simulink model "Cycle_model"  (R2024b)
settings: Solver=FixedStepAuto  StartTime=0.0  StopTime=300  FixedStep=0.01  RelTol=1e-3
InitFcn:
  | load matlab.mat
StopFcn:
  | startLoc = get_param(bdroot, 'ModelWorkspace').getVariable('startLoc');
  | assignin('base', 'startLoc', startLoc);
  | 
  | goalLoc = get_param(bdroot, 'ModelWorkspace').getVariable('goalLoc');
  | assignin('base', 'goalLoc', goalLoc);
  | 
  | InitState = get_param(bdroot, 'ModelWorkspace').getVariable('InitState');
  | assignin('base', 'InitState', InitState);
  | 
  | visualizador_datos_sim
model workspace (MAT data in the model file):
  InitState = [5 5 3.14159265359]
  Ts = 0.01
  goalLoc = [13 7]
  speed_range = [-8 8]
  startLoc = [5 5]
values from neighbouring files (symbols this model uses):
  simpleMap = [1 1 1 1 1 1 1 1 1 1 1 1 ... (702 elements, 26x27)]    [matlab.mat]
undefined symbols (not defined in the file or in its folder): dspblkCoreblockFVToolHelper, gcbh
libraries: simulink x5, slpidlib x2, robotmobilelib x1, robotalgslib x1
settings Model: Creator=Andres  LastModifiedBy=Andres
settings OptimizationCC: DefaultParameterBehavior=Inlined  GainParamInheritBuiltInType=on  UseFloatMulNetSlope=on  OptimizeBlockIOStorage=off
settings RTWCC: BuildConfiguration=Debug
settings CodeAppCC: ForceParamTrailComments=on  MATLABSourceComments=on

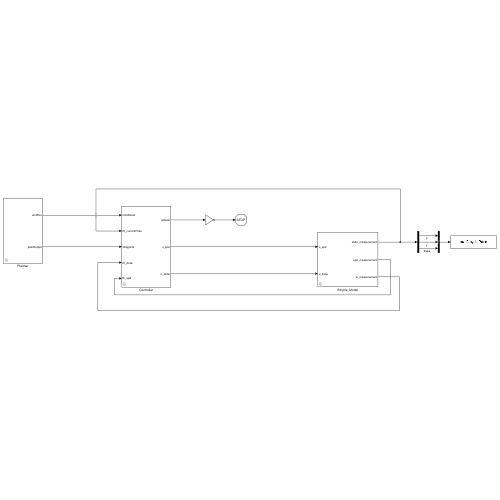
[thumbnail: Simulink's stored preview of the top-level diagram]
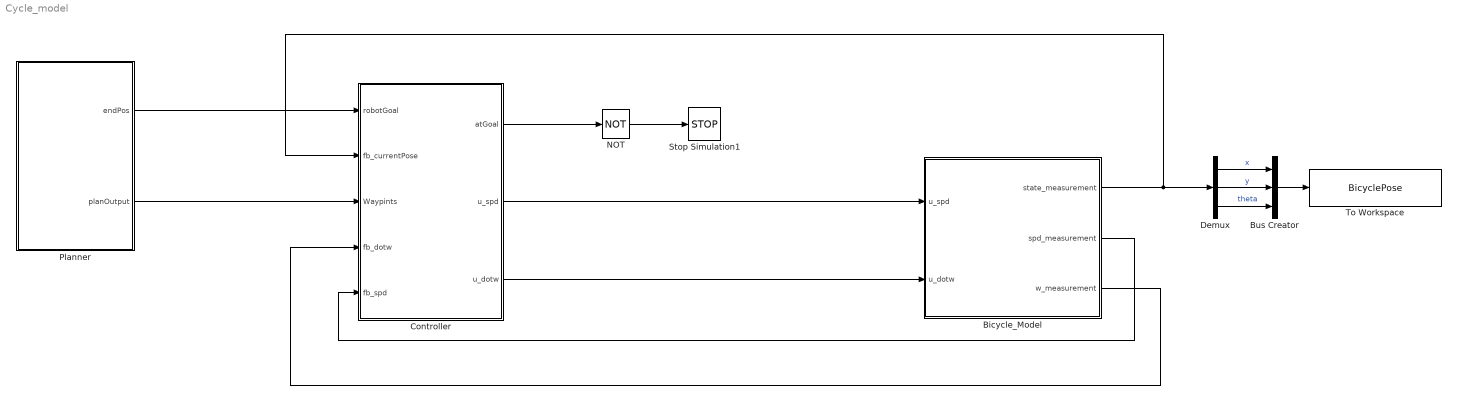
== system Cycle_model ==
  Bicycle_Model : Subsystem  mask{WheelBase=1, InitialState=InitState, MaxSteeringAngle=pi/4, VehicleSpeedRange=speed_range, tau_rad=0.2, tau_spd=3}
      mask prompts: WheelBase "robotics:robotslmobile:sharedblockmask:WheelBasePrompt"; InitialState "robotics:robotslmobile:sharedblockmask:InitialStatePrompt"; MaxSteeringAngle "robotics:robotslmobile:sharedblockmask:MaxSteeringAnglePrompt"; VehicleSpeedRange "robotics:robotslmobile:sharedblockmask:VehicleSpeedRangePrompt"; tau_rad "Time from 0 rad to max steering angle (s)"; tau_spd "Time form 0 m/s to max speed (s)"
      mask TypeOptions WheelBase: Model/WheelBase
      mask TypeOptions InitialState: Model/InitialState
      mask TypeOptions MaxSteeringAngle: Model/MaxSteeringAngle
      mask TypeOptions VehicleSpeedRange: Model/VehicleSpeedRange
      mask TypeOptions tau_rad: Model/tau_rad
      mask TypeOptions tau_spd: Model/tau_spd
      mask DialogControl DescGroupVar Prompt: Bicycle Model (mask)
      mask DialogControl WheelBase Prompt: Wheel base (m):
      mask DialogControl InitialState Prompt: Initial state:
      mask DialogControl MaxSteeringAngle Prompt: Maximum steering angle (rad):
      mask DialogControl VehicleSpeedRange Prompt: Vehicle speed range (m/s):
  Bus Creator : BusCreator  Inputs=3
  Controller : Subsystem  mask{Kp_dotw=1, Ki_dotw=0.01, Kp_lin=0.1, Ki_lin=0.1, DesiredLinearVelocity=2, LookaheadDistance=0.5, MaxAngularVelocity=7}
      mask prompts: Kp_dotw "Kp"; Ki_dotw "Ki"; Kp_lin "Kp"; Ki_lin "Ki"; DesiredLinearVelocity "Desired linear velocity (m/s):"; LookaheadDistance "Lookahead distance (m):"; MaxAngularVelocity "Maximum angular velocity (rad/s):"
      mask TypeOptions DesiredLinearVelocity: Pure Pursuit/DesiredLinearVelocity
      mask TypeOptions LookaheadDistance: Pure Pursuit/LookaheadDistance
      mask TypeOptions MaxAngularVelocity: Pure Pursuit/MaxAngularVelocity
      mask DialogControl DescGroupVar Prompt: Controller (mask)
      mask DialogControl ParameterGroupVar Prompt: PI angular velocity
      mask DialogControl ParameterGroupVar_copy Prompt: PI linear velocity
  Demux : Demux  Outputs=3
  NOT : Logic  Operator=NOT  IconShape=distinctive  AllPortsSameDT=off  OutDataTypeStr=boolean
  Planner : Subsystem  mask{startLoc=startLoc, goalLoc=goalLoc, simpleMap=simpleMap}
      mask prompts: startLoc "Start Location [x y]"; goalLoc "Goal Location"; simpleMap "Map"
      mask DialogControl DescGroupVar Prompt: Planner (mask)
  Stop Simulation1 : Stop
  To Workspace : ToWorkspace  VariableName=BicyclePose  SaveFormat=Timeseries  SampleTime=-1
  wires:
  NOT/1 -> Stop Simulation1/1
  Demux/1 -> Bus Creator/1  "x"
  Demux/2 -> Bus Creator/2  "y"
  Demux/3 -> Bus Creator/3  "theta"
  Bus Creator/1 -> To Workspace/1
  Bicycle_Model/1(state_measurement) -> Demux/1, Controller/2(fb_currentPose)
  Bicycle_Model/2(spd_measurement) -> Controller/5(fb_spd)
  Planner/1(endPos) -> Controller/1(robotGoal)
  Planner/2(planOutput) -> Controller/3(Waypints)
  Bicycle_Model/3(w_measurement) -> Controller/4(fb_dotw)
  Controller/1(atGoal) -> NOT/1
  Controller/2(u_spd) -> Bicycle_Model/1(u_spd)
  Controller/3(u_dotw) -> Bicycle_Model/2(u_dotw)

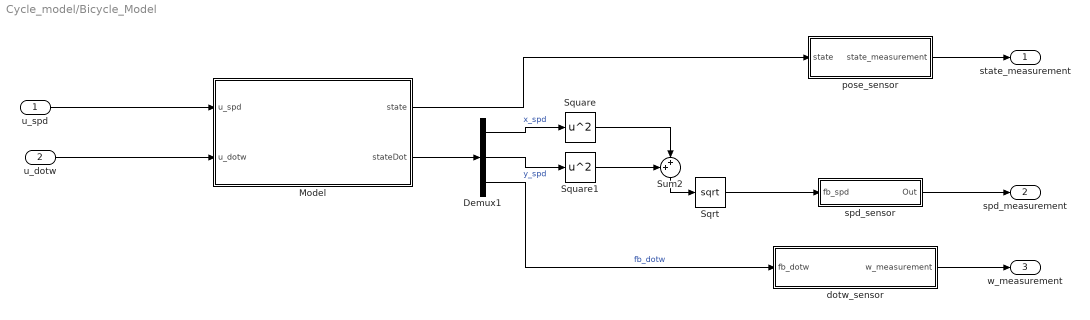
== system Cycle_model/Bicycle_Model ==
  u_spd : Inport
  u_dotw : Inport  Port=2
  Demux1 : Demux  Outputs=3
  Model : Subsystem  mask{InitialState=InitialState, WheelBase=WheelBase, VehicleSpeedRange=VehicleSpeedRange, MaxSteeringAngle=MaxSteeringAngle, tau_spd=tau_spd, tau_rad=tau_rad}
      mask prompts: InitialState "robotics:robotslmobile:sharedblockmask:InitialStatePrompt"; WheelBase "robotics:robotslmobile:sharedblockmask:WheelBasePrompt"; VehicleSpeedRange "robotics:robotslmobile:sharedblockmask:VehicleSpeedRangePrompt"; MaxSteeringAngle "robotics:robotslmobile:sharedblockmask:MaxSteeringAnglePrompt"; tau_spd "Time form 0 m/s to max speed (s)"; tau_rad "Time from 0 rad to max steering angle (s)"
      mask TypeOptions InitialState: Bicycle Kinematic Model/InitialState
      mask TypeOptions WheelBase: Bicycle Kinematic Model/WheelBase
      mask TypeOptions VehicleSpeedRange: Bicycle Kinematic Model/VehicleSpeedRange
      mask TypeOptions MaxSteeringAngle: Bicycle Kinematic Model/MaxSteeringAngle
      mask DialogControl ParameterGroupVar Prompt: Bicycle Parameters
      mask DialogControl InitialState Prompt: Initial state:
      mask DialogControl WheelBase Prompt: Wheel base (m):
      mask DialogControl VehicleSpeedRange Prompt: Vehicle speed range (m/s):
      mask DialogControl MaxSteeringAngle Prompt: Maximum steering angle (rad):
  Sqrt : Sqrt
  Square : Math  Operator=square
  Square1 : Math  Operator=square
  Sum2 : Sum  Inputs=++|
  dotw_sensor : Subsystem
  pose_sensor : Subsystem
  spd_sensor : Subsystem  mask{NsPw=0.0000004, Nhz=1000}
      mask prompts: NsPw "Noise Power"; Nhz "Noise Hz"
  state_measurement : Outport
  spd_measurement : Outport  Port=2
  w_measurement : Outport  Port=3
  wires:
  Square1/1 -> Sum2/1
  Demux1/1 -> Square/1  "x_spd"
  Sqrt/1 -> spd_sensor/1(fb_spd)
  Demux1/2 -> Square1/1  "y_spd"
  Model/2(stateDot) -> Demux1/1
  Square/1 -> Sum2/2
  Sum2/1 -> Sqrt/1
  u_dotw/1 -> Model/2(u_dotw)
  u_spd/1 -> Model/1(u_spd)
  Demux1/3 -> dotw_sensor/1(fb_dotw)  "fb_dotw"
  Model/1(state) -> pose_sensor/1(state)
  pose_sensor/1(state_measurement) -> state_measurement/1
  spd_sensor/1(Out) -> spd_measurement/1
  dotw_sensor/1(w_measurement) -> w_measurement/1

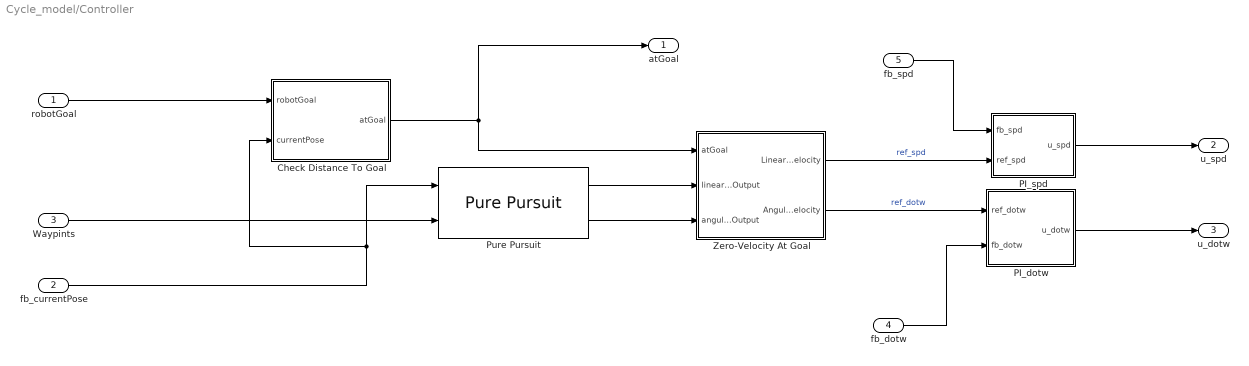
== system Cycle_model/Controller ==
  robotGoal : Inport
  fb_currentPose : Inport  Port=2
  Waypints : Inport  Port=3
  fb_dotw : Inport  Port=4
  fb_spd : Inport  Port=5
  Check Distance To Goal : Subsystem
  PI_dotw : Subsystem
  PI_spd : Subsystem
  Pure Pursuit : robotalgslib/Pure Pursuit  DesiredLinearVelocityPort=off  DesiredLinearVelocity=DesiredLinearVelocity  MaxAngularVelocity=MaxAngularVelocity  LookaheadDistancePort=off  LookaheadDistance=LookaheadDistance  TargetDirPort=off  SimulateUsing=Code generation
      settings: LibrarySourceBlock=robotmobilelib/Pure Pursuit
  Zero-Velocity At Goal : Subsystem
  atGoal : Outport
  u_spd : Outport  Port=2
  u_dotw : Outport  Port=3
  wires:
  Pure Pursuit/2 -> Zero-Velocity At Goal/3(angularVelocityOutput)
  Pure Pursuit/1 -> Zero-Velocity At Goal/2(linearVelocityOutput)
  fb_currentPose/1 -> Pure Pursuit/1, Check Distance To Goal/2(currentPose)
  Check Distance To Goal/1(atGoal) -> atGoal/1, Zero-Velocity At Goal/1(atGoal)
  fb_spd/1 -> PI_spd/1(fb_spd)
  fb_dotw/1 -> PI_dotw/2(fb_dotw)
  robotGoal/1 -> Check Distance To Goal/1(robotGoal)
  Waypints/1 -> Pure Pursuit/2
  Zero-Velocity At Goal/2(Angular Velocity) -> PI_dotw/1(ref_dotw)  "ref_dotw"
  PI_dotw/1(u_dotw) -> u_dotw/1
  PI_spd/1(u_spd) -> u_spd/1
  Zero-Velocity At Goal/1(Linear Velocity) -> PI_spd/2(ref_spd)  "ref_spd"

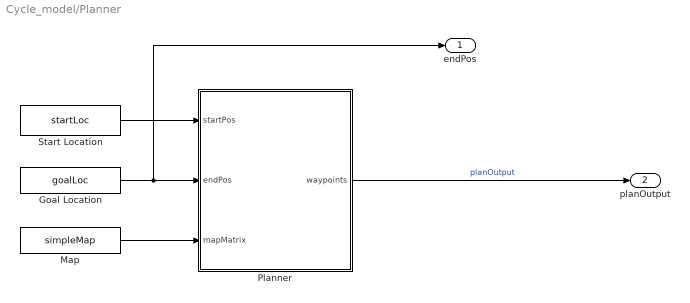
== system Cycle_model/Planner ==
  Goal Location : Constant  Value=goalLoc
  Map : Constant  Value=simpleMap
  Planner : MATLAB Function  TreatAsAtomicUnit=on
  Start Location : Constant  Value=startLoc
  endPos : Outport
  planOutput : Outport  Port=2
  wires:
  Goal Location/1 -> endPos/1, Planner/2(endPos)
  Start Location/1 -> Planner/1(startPos)
  Map/1 -> Planner/3(mapMatrix)
  Planner/1(waypoints) -> planOutput/1  "planOutput"

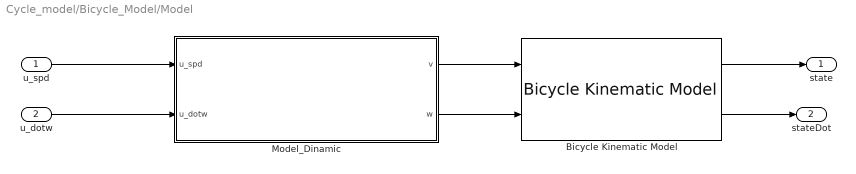
== system Cycle_model/Bicycle_Model/Model ==
  u_spd : Inport
  u_dotw : Inport  Port=2
  Bicycle Kinematic Model : robotmobilelib/Bicycle Kinematic Model  VehicleInputs=Vehicle Speed & Heading Angular Velocity  WheelBase=WheelBase  VehicleSpeedRange=VehicleSpeedRange  MaxSteeringAngle=MaxSteeringAngle  InitialState=InitialState  SimulateUsing=Interpreted execution
  Model_Dinamic : Subsystem
  state : Outport
  stateDot : Outport  Port=2
  wires:
  Bicycle Kinematic Model/1 -> state/1
  Bicycle Kinematic Model/2 -> stateDot/1
  u_spd/1 -> Model_Dinamic/1(u_spd)
  Model_Dinamic/1(v) -> Bicycle Kinematic Model/1
  Model_Dinamic/2(w) -> Bicycle Kinematic Model/2
  u_dotw/1 -> Model_Dinamic/2(u_dotw)

== system Cycle_model/Bicycle_Model/dotw_sensor ==
  fb_dotw : Inport
  Low-Pass Filter1 : TransferFcn  Denominator=[0.05 1]
  Zero-Order Hold3 : ZeroOrderHold  SampleTime=Ts
  w_measurement : Outport
  wires:
  Low-Pass Filter1/1 -> Zero-Order Hold3/1
  Zero-Order Hold3/1 -> w_measurement/1
  fb_dotw/1 -> Low-Pass Filter1/1

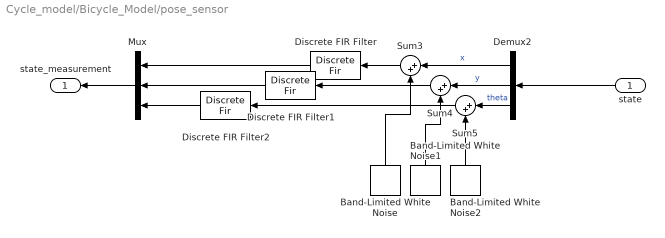
== system Cycle_model/Bicycle_Model/pose_sensor ==
  state : Inport
  Band-Limited White Noise : simulink/Sources/Band-Limited White Noise  Cov=[0.0004]  Ts=0.1  seed=123
  Band-Limited White Noise1 : simulink/Sources/Band-Limited White Noise  Cov=[0.0004]  Ts=0.1  seed=456
  Band-Limited White Noise2 : simulink/Sources/Band-Limited White Noise  Cov=0.000025  Ts=0.1  seed=789
  Demux2 : Demux  Outputs=3
  Discrete FIR Filter : DiscreteFir  LoadFcn=dspblkCoreblockFVToolHelper(gcbh,'load');  Coefficients="[0.0625,  0.2500,  0.3750,  0.2500,  0.0625]"  InitialStates=5
      settings: CopyFcn=dspblkCoreblockFVToolHelper(gcbh,'copy');  DeleteFcn=dspblkCoreblockFVToolHelper(gcbh,'close');  ModelCloseFcn=dspblkCoreblockFVToolHelper(gcbh,'close');  PreSaveFcn=dspblkCoreblockFVToolHelper(gcbh,'presave');  PostSaveFcn=dspblkCoreblockFVToolHelper(gcbh,'postsave');  CloseFcn=dspblkCoreblockFVToolHelper(gcbh,'close');
  Discrete FIR Filter1 : DiscreteFir  LoadFcn=dspblkCoreblockFVToolHelper(gcbh,'load');  Coefficients="[0.0625,  0.2500,  0.3750,  0.2500,  0.0625]"  InitialStates=5
      settings: CopyFcn=dspblkCoreblockFVToolHelper(gcbh,'copy');  DeleteFcn=dspblkCoreblockFVToolHelper(gcbh,'close');  ModelCloseFcn=dspblkCoreblockFVToolHelper(gcbh,'close');  PreSaveFcn=dspblkCoreblockFVToolHelper(gcbh,'presave');  PostSaveFcn=dspblkCoreblockFVToolHelper(gcbh,'postsave');  CloseFcn=dspblkCoreblockFVToolHelper(gcbh,'close');
  Discrete FIR Filter2 : DiscreteFir  LoadFcn=dspblkCoreblockFVToolHelper(gcbh,'load');  Coefficients="[0.0625,  0.2500,  0.3750,  0.2500,  0.0625]"  InitialStates=pi
      settings: CopyFcn=dspblkCoreblockFVToolHelper(gcbh,'copy');  DeleteFcn=dspblkCoreblockFVToolHelper(gcbh,'close');  ModelCloseFcn=dspblkCoreblockFVToolHelper(gcbh,'close');  PreSaveFcn=dspblkCoreblockFVToolHelper(gcbh,'presave');  PostSaveFcn=dspblkCoreblockFVToolHelper(gcbh,'postsave');  CloseFcn=dspblkCoreblockFVToolHelper(gcbh,'close');
  Mux : Mux  Inputs=3
  Sum3 : Sum  Inputs=|++
  Sum4 : Sum  Inputs=|++
  Sum5 : Sum  Inputs=|++
  state_measurement : Outport
  wires:
  Sum4/1 -> Discrete FIR Filter1/1
  Band-Limited White Noise/1 -> Sum3/2
  Sum5/1 -> Discrete FIR Filter2/1
  Discrete FIR Filter/1 -> Mux/1
  Demux2/2 -> Sum4/1  "y"
  Band-Limited White Noise1/1 -> Sum4/2
  Discrete FIR Filter1/1 -> Mux/2
  Band-Limited White Noise2/1 -> Sum5/2
  Discrete FIR Filter2/1 -> Mux/3
  Demux2/3 -> Sum5/1  "theta"
  Sum3/1 -> Discrete FIR Filter/1
  Demux2/1 -> Sum3/1  "x"
  Mux/1 -> state_measurement/1
  state/1 -> Demux2/1

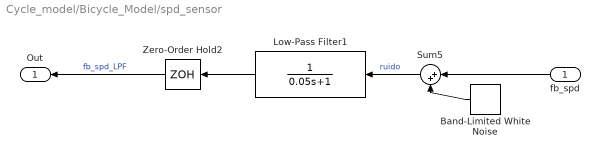
== system Cycle_model/Bicycle_Model/spd_sensor ==
  fb_spd : Inport
  Band-Limited White Noise : simulink/Sources/Band-Limited White Noise  Cov=[NsPw]  Ts=Ts  seed=[23341]
  Low-Pass Filter1 : TransferFcn  Denominator=[0.05 1]
  Sum5 : Sum  Inputs=|++
  Zero-Order Hold2 : ZeroOrderHold  SampleTime=Ts
  Out : Outport
  wires:
  Low-Pass Filter1/1 -> Zero-Order Hold2/1
  Sum5/1 -> Low-Pass Filter1/1  "ruido"
  Band-Limited White Noise/1 -> Sum5/2
  fb_spd/1 -> Sum5/1
  Zero-Order Hold2/1 -> Out/1  "fb_spd_LPF"

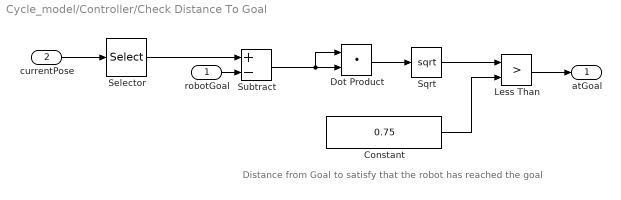
== system Cycle_model/Controller/Check Distance To Goal ==
  note: Distance from Goal to satisfy that the robot has reached the goal
  robotGoal : Inport
  currentPose : Inport  Port=2
  Constant : Constant  Value=0.75
  Dot Product : DotProduct  OutDataTypeStr=Inherit: Inherit via internal rule
  Less Than : RelationalOperator  Operator=>  OutDataTypeStr=boolean  RndMeth=Simplest  InputSameDT=off
  Selector : Selector  InputPortWidth=3  IndexOptions=Index vector (dialog)  Indices=[1 2]  OutputSizes=1
  Sqrt : Sqrt
  Subtract : Sum  Inputs=+-
  atGoal : Outport
  wires:
  robotGoal/1 -> Subtract/2
  Dot Product/1 -> Sqrt/1
  Constant/1 -> Less Than/2
  currentPose/1 -> Selector/1
  Less Than/1 -> atGoal/1
  Sqrt/1 -> Less Than/1
  Subtract/1 -> Dot Product/1, Dot Product/2
  Selector/1 -> Subtract/1

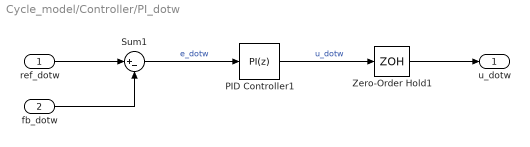
== system Cycle_model/Controller/PI_dotw ==
  ref_dotw : Inport
  fb_dotw : Inport  Port=2
  PID Controller1 : slpidlib/PID Controller  Controller=PI  Form=Parallel  TimeDomain=Discrete-time  UseExternalTs=off  SampleTime=Ts  IntegratorMethod=Forward Euler  FilterMethod=Forward Euler  ControllerParametersSource=internal  P=Kp_dotw  I=Ki_dotw  UseKiTs=off  D=0  UseExternalDerivativeSource=off  N=100  UseFilter=on  TunerSelectOption=Transfer Function Based (PID Tuner App)  InitialConditionSource=internal  InitialConditionForIntegrator=0  InitialConditionForFilter=0  DifferentiatorICPrevScaledInput=0  ExternalReset=none  TrackingMode=off  Kt=1  LimitOutput=on  SatLimitsSource=internal  UpperSaturationLimit=1  LowerSaturationLimit=-1  LinearizeAsGain=off  AntiWindupMode=clamping  Kb=0.01  LimitIntegrator=off  UpperIntegratorSaturationLimit=inf  LowerIntegratorSaturationLimit=-inf  POutMin=[]  POutMax=[]  IOutMin=[]  IOutMax=[]  DOutMin=[]  DOutMax=[]  NOutMin=[]  NOutMax=[]  SumOutMin=[]  SumOutMax=[]  SaturationOutMin=[]  SaturationOutMax=[]  PParamMin=[]  PParamMax=[]  IParamMin=[]  IParamMax=[]  DParamMin=[]  DParamMax=[]  NParamMin=[]  NParamMax=[]  KbParamMin=[]  KbParamMax=[]  KtParamMin=[]  KtParamMax=[]  KbOutMin=[]  KbOutMax=[]  KtOutMin=[]  KtOutMax=[]  IntegratorOutMin=[]  IntegratorOutMax=[]  FilterOutMin=[]  FilterOutMax=[]  SumI1OutMin=[]  SumI1OutMax=[]  SumI2OutMin=[]  SumI2OutMax=[]  SumI3OutMin=[]  SumI3OutMax=[]  SumI4OutMin=[]  SumI4OutMax=[]  SumDOutMin=[]  SumDOutMax=[]  DifferentiatorOutMin=[]  DifferentiatorOutMax=[]  FilterDiffOutCoefMin=[]  FilterDiffOutCoefMax=[]  ReciprocalOutMin=[]  ReciprocalOutMax=[]  SumDenOutMin=[]  SumDenOutMax=[]  SumNumOutMin=[]  SumNumOutMax=[]  DivideOutMin=[]  DivideOutMax=[]  UdiffTsProdOutMin=[]  UdiffTsProdOutMax=[]  NTsProdOutMin=[]  NTsProdOutMax=[]  UintegralTsProdOutMin=[]  UintegralTsProdOutMax=[]  UngainTsProdOutMin=[]  UngainTsProdOutMax=[]  ClampingZeroOutDataTypeStr=Inherit: Inherit via back propagation  ClampingZeroOutMin=[]  ClampingZeroOutMax=[]  FilterDenConstantOutDataTypeStr=Inherit: Inherit via back propagation  FilterDenConstantOutMin=[]  FilterDenConstantOutMax=[]  PCopyOutDataTypeStr=Inherit: Inherit via back propagation  PCopyOutMin=[]  PCopyOutMax=[]  NCopyOutDataTypeStr=Inherit: Inherit via back propagation  NCopyOutMin=[]  NCopyOutMax=[]  IntegratorContinuousStateAttributes=''  IntegratorStateMustResolveToSignalObject=off  IntegratorRTWStateStorageClass=Auto  FilterContinuousStateAttributes=''  FilterStateMustResolveToSignalObject=off  FilterRTWStateStorageClass=Auto  ParallelPVariant=InternalParameters  IdealPVariant=Disabled  IVariant=InternalParameters  DVariant=Disabled  IntegratorVariant=Discrete  SatVariant=Enabled  AWVariant=DiscClampingParallel  PCopyVariant=Disabled  TRVariant=Disabled  FdbkBlocksVariant=Forward  IdealPFdbkVariant=Disabled  SatFdbkVariant=Disabled  DerivativeFilterVariant=Disabled  NVariant=Disabled  NCopyVariant=Disabled_SignalSpec  FilterICVariant=Disabled  IntegratorICVariant=InternalICs  ExternalResetVariant=Disabled  TRSumVariant=Passthrough  SumFdbkVariant=Disabled  SumVariant=Sum_PI  TsampFilterVariant=InternalTs  TsampNgainVariant=Passthrough  TsampIntegralVariant=Disabled_SignalSpec  ExternalSaturationOutDataTypeStr=Inherit: Same as second input  DerivativeSourceVariant=Disabled  PreIntVariant=InternalPreInt
  Sum1 : Sum  Inputs=|+-
  Zero-Order Hold1 : ZeroOrderHold  SampleTime=Ts
  u_dotw : Outport
  wires:
  Sum1/1 -> PID Controller1/1  "e_dotw"
  PID Controller1/1 -> Zero-Order Hold1/1  "u_dotw"
  Zero-Order Hold1/1 -> u_dotw/1
  ref_dotw/1 -> Sum1/1
  fb_dotw/1 -> Sum1/2

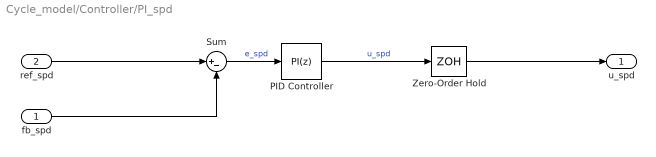
== system Cycle_model/Controller/PI_spd ==
  fb_spd : Inport
  ref_spd : Inport  Port=2
  PID Controller : slpidlib/PID Controller  Controller=PI  Form=Parallel  TimeDomain=Discrete-time  UseExternalTs=off  SampleTime=Ts  IntegratorMethod=Forward Euler  FilterMethod=Forward Euler  ControllerParametersSource=internal  P=Kp_lin  I=Ki_lin  UseKiTs=off  D=0  UseExternalDerivativeSource=off  N=100  UseFilter=on  TunerSelectOption=Transfer Function Based (PID Tuner App)  InitialConditionSource=internal  InitialConditionForIntegrator=0  InitialConditionForFilter=0  DifferentiatorICPrevScaledInput=0  ExternalReset=none  TrackingMode=off  Kt=1  LimitOutput=on  SatLimitsSource=internal  UpperSaturationLimit=1  LowerSaturationLimit=-1  LinearizeAsGain=on  AntiWindupMode=clamping  Kb=0.01  LimitIntegrator=off  UpperIntegratorSaturationLimit=inf  LowerIntegratorSaturationLimit=-inf  POutMin=[]  POutMax=[]  IOutMin=[]  IOutMax=[]  DOutMin=[]  DOutMax=[]  NOutMin=[]  NOutMax=[]  SumOutMin=[]  SumOutMax=[]  SaturationOutMin=[]  SaturationOutMax=[]  PParamMin=[]  PParamMax=[]  IParamMin=[]  IParamMax=[]  DParamMin=[]  DParamMax=[]  NParamMin=[]  NParamMax=[]  KbParamMin=[]  KbParamMax=[]  KtParamMin=[]  KtParamMax=[]  KbOutMin=[]  KbOutMax=[]  KtOutMin=[]  KtOutMax=[]  IntegratorOutMin=[]  IntegratorOutMax=[]  FilterOutMin=[]  FilterOutMax=[]  SumI1OutMin=[]  SumI1OutMax=[]  SumI2OutMin=[]  SumI2OutMax=[]  SumI3OutMin=[]  SumI3OutMax=[]  SumI4OutMin=[]  SumI4OutMax=[]  SumDOutMin=[]  SumDOutMax=[]  DifferentiatorOutMin=[]  DifferentiatorOutMax=[]  FilterDiffOutCoefMin=[]  FilterDiffOutCoefMax=[]  ReciprocalOutMin=[]  ReciprocalOutMax=[]  SumDenOutMin=[]  SumDenOutMax=[]  SumNumOutMin=[]  SumNumOutMax=[]  DivideOutMin=[]  DivideOutMax=[]  UdiffTsProdOutMin=[]  UdiffTsProdOutMax=[]  NTsProdOutMin=[]  NTsProdOutMax=[]  UintegralTsProdOutMin=[]  UintegralTsProdOutMax=[]  UngainTsProdOutMin=[]  UngainTsProdOutMax=[]  ClampingZeroOutDataTypeStr=Inherit: Inherit via back propagation  ClampingZeroOutMin=[]  ClampingZeroOutMax=[]  FilterDenConstantOutDataTypeStr=Inherit: Inherit via back propagation  FilterDenConstantOutMin=[]  FilterDenConstantOutMax=[]  PCopyOutDataTypeStr=Inherit: Inherit via back propagation  PCopyOutMin=[]  PCopyOutMax=[]  NCopyOutDataTypeStr=Inherit: Inherit via back propagation  NCopyOutMin=[]  NCopyOutMax=[]  IntegratorContinuousStateAttributes=''  IntegratorStateMustResolveToSignalObject=off  IntegratorRTWStateStorageClass=Auto  FilterContinuousStateAttributes=''  FilterStateMustResolveToSignalObject=off  FilterRTWStateStorageClass=Auto  ParallelPVariant=InternalParameters  IdealPVariant=Disabled  IVariant=InternalParameters  DVariant=Disabled  IntegratorVariant=Discrete  SatVariant=Enabled  AWVariant=DiscClampingParallel  PCopyVariant=Disabled  TRVariant=Disabled  FdbkBlocksVariant=Forward  IdealPFdbkVariant=Disabled  SatFdbkVariant=Disabled  DerivativeFilterVariant=Disabled  NVariant=Disabled  NCopyVariant=Disabled_SignalSpec  FilterICVariant=Disabled  IntegratorICVariant=InternalICs  ExternalResetVariant=Disabled  TRSumVariant=Passthrough  SumFdbkVariant=Disabled  SumVariant=Sum_PI  TsampFilterVariant=InternalTs  TsampNgainVariant=Passthrough  TsampIntegralVariant=Disabled_SignalSpec  ExternalSaturationOutDataTypeStr=Inherit: Same as second input  DerivativeSourceVariant=Disabled  PreIntVariant=InternalPreInt
  Sum : Sum  Inputs=|+-
  Zero-Order Hold : ZeroOrderHold  SampleTime=Ts
  u_spd : Outport
  wires:
  Sum/1 -> PID Controller/1  "e_spd"
  ref_spd/1 -> Sum/1
  fb_spd/1 -> Sum/2
  PID Controller/1 -> Zero-Order Hold/1  "u_spd"
  Zero-Order Hold/1 -> u_spd/1

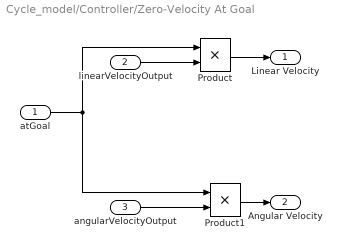
== system Cycle_model/Controller/Zero-Velocity At Goal ==
  atGoal : Inport
  linearVelocityOutput : Inport  Port=2
  angularVelocityOutput : Inport  Port=3
  Product : Product
  Product1 : Product
  Linear Velocity : Outport  OutDataTypeStr=double
  Angular Velocity : Outport  Port=2  OutDataTypeStr=double
  wires:
  atGoal/1 -> Product1/1, Product/1
  angularVelocityOutput/1 -> Product1/2
  linearVelocityOutput/1 -> Product/2
  Product/1 -> Linear Velocity/1
  Product1/1 -> Angular Velocity/1

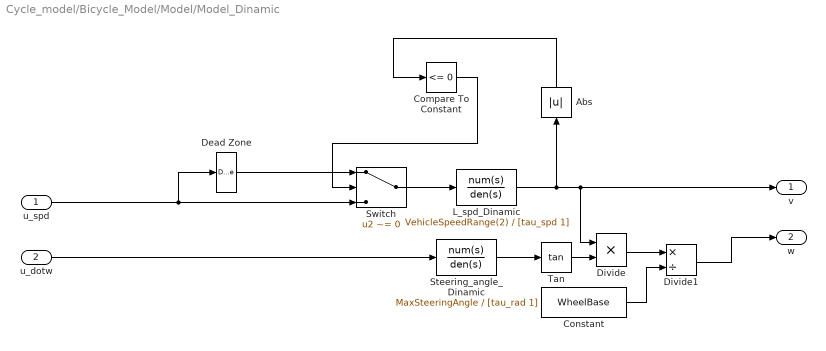
== system Cycle_model/Bicycle_Model/Model/Model_Dinamic ==
  u_spd : Inport
  u_dotw : Inport  Port=2
  Abs : Abs  SaturateOnIntegerOverflow=off
  Compare To Constant : simulink/Logic and Bit Operations/Compare To Constant  relop=<=  const=0  OutDataTypeStr=boolean
  Constant : Constant  Value=WheelBase
  Dead Zone : DeadZone  LowerValue=-0.25  UpperValue=0.25
  Divide : Product  Inputs=**
  Divide1 : Product  Inputs=*/
  L_spd_Dinamic : TransferFcn  Numerator=VehicleSpeedRange(2)  Denominator=[tau_spd 1]
  Steering_angle_Dinamic : TransferFcn  Numerator=MaxSteeringAngle  Denominator=[tau_rad 1]
  Switch : Switch  Criteria=u2 ~= 0  SaturateOnIntegerOverflow=off  InputSameDT=off
  Tan : Trigonometry  Operator=tan
  v : Outport
  w : Outport  Port=2
  wires:
  Dead Zone/1 -> Switch/1
  Steering_angle_Dinamic/1 -> Tan/1
  Constant/1 -> Divide1/2
  L_spd_Dinamic/1 -> Abs/1, v/1, Divide/1
  Abs/1 -> Compare To Constant/1
  Divide/1 -> Divide1/1
  u_spd/1 -> Dead Zone/1, Switch/3
  Tan/1 -> Divide/2
  Compare To Constant/1 -> Switch/2
  Switch/1 -> L_spd_Dinamic/1
  Divide1/1 -> w/1
  u_dotw/1 -> Steering_angle_Dinamic/1

== matlab function Cycle_model/Planner/Planner ==
  settings: updateMethod=DISCRETE
  data: startPos input size=[1 2]; endPos input size=[1 2]; waypoints output size=[100 2]; mapMatrix input
function waypoints = planning(startPos, endPos, mapMatrix)

persistent waypointsInternal
persistent prevStartPos
persistent prevEndPos

% Set constant parameters
maxNumNodes = 100;

% Initialize persistent variables that are used downstream
if isempty(prevStartPos)
    prevStartPos = startPos;
end

if isempty(prevEndPos)
    prevEndPos = endPos;
end

isNewPath = (~isequal(prevStartPos, startPos) || ~isequal(prevEndPos, endPos));

if isempty(waypointsInternal) || isNewPath
    % Two conditions in which waypoints must be set: they are not yet
    % initialized, or they are initialized, but the current start and end
    % do not match those used to generate the previous set of waypoints
    [waypointsInternal] = planPath(mapMatrix, maxNumNodes, startPos, endPos);
end

% Update the outputs
waypoints = waypointsInternal;

% Update the persistent variables that indicate previous state
prevStartPos = startPos;
prevEndPos = endPos;

%% Helper Function

function wayPoints = planPath(mapMatrix, maxNodes, startPos, endPos)
    
    % Create a probabilistic roadmap
    map = binaryOccupancyMap(mapMatrix);
    prm = mobileRobotPRM(map, maxNodes);
    
    % Find a path between two points
    xy = findpath(prm, startPos, endPos);
    wayPoints = repmat(endPos, maxNodes, 1);
    
    % Number of nodes that are actually used
    numNodes = length(xy);
    wayPoints(1:numNodes,:) = xy;    

end

end
